simulink model "tut2_4"  (R2018b)
settings: Solver=VariableStepAuto  StartTime=0.0  StopTime=10.0  RelTol=1e-3
values from neighbouring files (symbols this model uses):
  C_inf = evalfr(C, inf)    [tut2.m]
libraries: cstblocks x6
settings Model: Creator=c3277928  LastModifiedBy=c3277928

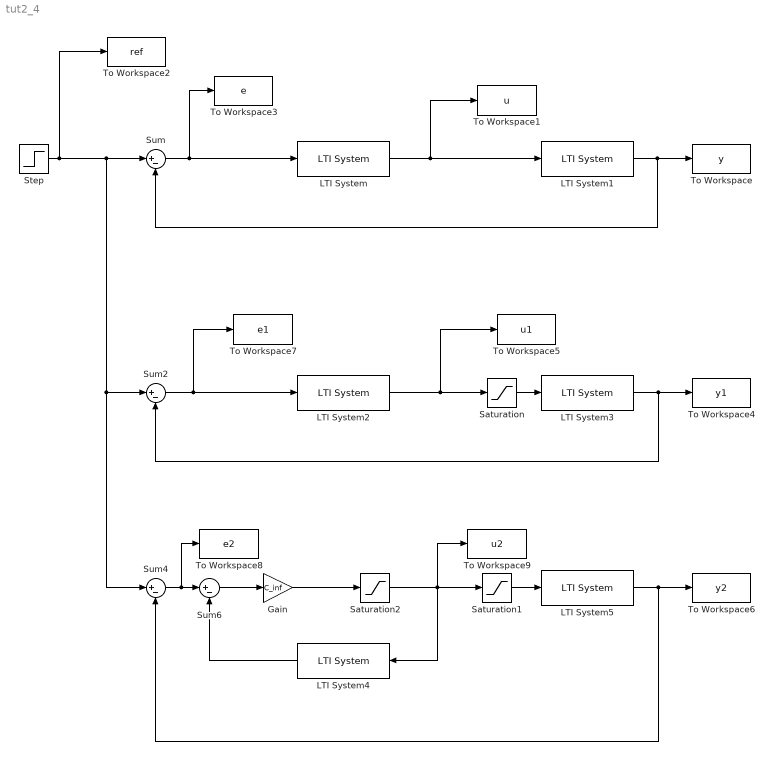
== system tut2_4 ==
  Gain : Gain  Gain=C_inf
  LTI System : cstblocks/LTI System  sys=C  IC=[]
  LTI System1 : cstblocks/LTI System  sys=G0  IC=[]
  LTI System2 : cstblocks/LTI System  sys=C  IC=[]
  LTI System3 : cstblocks/LTI System  sys=G0  IC=[]
  LTI System4 : cstblocks/LTI System  sys=C_feedback  IC=[]
  LTI System5 : cstblocks/LTI System  sys=G0  IC=[]
  Saturation : Saturate  UpperLimit=2  LowerLimit=-2
  Saturation1 : Saturate  UpperLimit=2  LowerLimit=-2
  Saturation2 : Saturate  UpperLimit=2  LowerLimit=-2
  Step : Step  Time=0  SampleTime=0
  Sum{,2,4,6} (4 alike) : Sum  Inputs=|+-
  To Workspace : ToWorkspace  VariableName=y  SaveFormat=Timeseries  SampleTime=-1
  To Workspace1 : ToWorkspace  VariableName=u  SaveFormat=Timeseries  SampleTime=-1
  To Workspace2 : ToWorkspace  VariableName=ref  SaveFormat=Timeseries  SampleTime=-1
  To Workspace3 : ToWorkspace  VariableName=e  SaveFormat=Timeseries  SampleTime=-1
  To Workspace4 : ToWorkspace  VariableName=y1  SaveFormat=Timeseries  SampleTime=-1
  To Workspace5 : ToWorkspace  VariableName=u1  SaveFormat=Timeseries  SampleTime=-1
  To Workspace6 : ToWorkspace  VariableName=y2  SaveFormat=Timeseries  SampleTime=-1
  To Workspace7 : ToWorkspace  VariableName=e1  SaveFormat=Timeseries  SampleTime=-1
  To Workspace8 : ToWorkspace  VariableName=e2  SaveFormat=Timeseries  SampleTime=-1
  To Workspace9 : ToWorkspace  VariableName=u2  SaveFormat=Timeseries  SampleTime=-1
  wires:
  LTI System/1 -> LTI System1/1, To Workspace1/1
  Sum6/1 -> Gain/1
  Gain/1 -> Saturation2/1
  Saturation2/1 -> To Workspace9/1, LTI System4/1, Saturation1/1
  Saturation/1 -> LTI System3/1
  Sum4/1 -> To Workspace8/1, Sum6/1
  LTI System1/1 -> To Workspace/1, Sum/2
  Saturation1/1 -> LTI System5/1
  LTI System2/1 -> To Workspace5/1, Saturation/1
  LTI System4/1 -> Sum6/2
  Step/1 -> Sum/1, Sum2/1, Sum4/1, To Workspace2/1
  LTI System5/1 -> To Workspace6/1, Sum4/2
  LTI System3/1 -> To Workspace4/1, Sum2/2
  Sum/1 -> LTI System/1, To Workspace3/1
  Sum2/1 -> To Workspace7/1, LTI System2/1
